simulink model "Ex_2"  (R2020a)
settings: Solver=VariableStepAuto  StartTime=0.0  StopTime=10.0  RelTol=1e-3
values from neighbouring files (symbols this model uses):
  A = [-1 0 0; -1 -2 -101; 1 1 0]    [Ex_1.m]
  A_d = ilaplace(H_s)    [Ex_1.m]
  B = [0 1; 1 -1; 0 0]    [Ex_1.m]
  B_d = int(A_d_tau * B, tau, 0, h)    [Ex_1.m]
  C = [1 0 101]    [Ex_1.m]
  C_d = C    [Ex_1.m]
  D = [0 0]    [Ex_1.m]
  D_d = D    [Ex_1.m]
  h = 0.01    [Ex_1.m]
undefined symbols (not defined in the file or in its folder): den1s, den1z, den2s, den2z, num1s, num1z, num2s, num2z
settings Model: Creator=Alexandru Olteanu  LastModifiedBy=Alexandru Olteanu

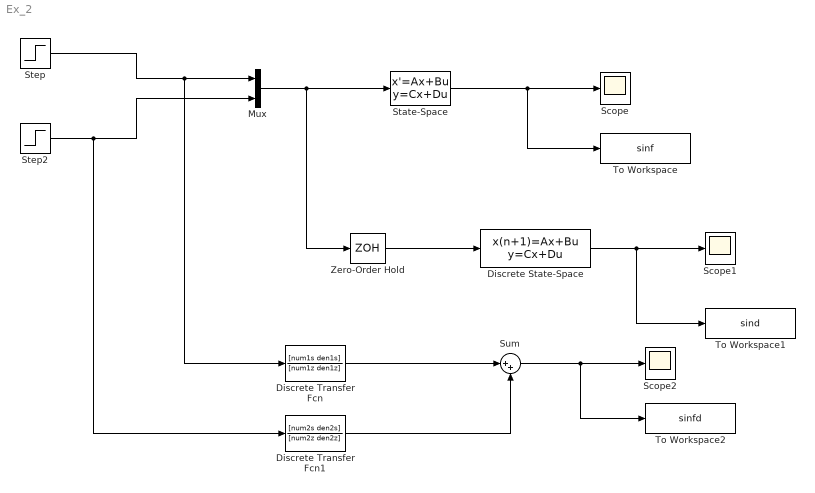
== system Ex_2 ==
  Discrete Transfer Fcn : DiscreteTransferFcn  Numerator=[num1s den1s]  Denominator=[num1z den1z]
  Discrete Transfer Fcn1 : DiscreteTransferFcn  Numerator=[num2s den2s]  Denominator=[num2z den2z]
  Discrete State-Space : DiscreteStateSpace  A=[A_d]  B=[B_d]  C=[C_d]  D=[D_d]  SampleTime=-1
  Mux : Mux  Inputs=2
  Scope : Scope
  Scope1 : Scope
  Scope2 : Scope
  State-Space : StateSpace  A=[A]  B=[B]  C=[C]  D=[D]  InitialCondition=0
  Step : Step  Time=0  SampleTime=0
  Step2 : Step  Time=0  After=-2  SampleTime=0
  Sum : Sum  Inputs=|++
  To Workspace : ToWorkspace  VariableName=sinf  SaveFormat=Timeseries  SampleTime=-1
  To Workspace1 : ToWorkspace  VariableName=sind  SaveFormat=Timeseries  SampleTime=-1
  To Workspace2 : ToWorkspace  VariableName=sinfd  SaveFormat=Timeseries  SampleTime=-1
  Zero-Order Hold : ZeroOrderHold  SampleTime=h
  wires:
  Step/1 -> Discrete Transfer Fcn/1, Mux/1
  Step2/1 -> Discrete Transfer Fcn1/1, Mux/2
  State-Space/1 -> To Workspace/1, Scope/1
  Mux/1 -> Zero-Order Hold/1, State-Space/1
  Zero-Order Hold/1 -> Discrete State-Space/1
  Discrete State-Space/1 -> To Workspace1/1, Scope1/1
  Discrete Transfer Fcn/1 -> Sum/1
  Discrete Transfer Fcn1/1 -> Sum/2
  Sum/1 -> To Workspace2/1, Scope2/1
